simulink model "zawieszenie_samochodu"  (R2021b)
settings: Solver=ode4  StartTime=0.0  StopTime=10.0  FixedStep=1/1000  RelTol=1e-3
values from neighbouring files (symbols this model uses):
  A = [0 0 1 0; 0 0 0 1; -(k1 + k2)/m1 k2/m1 -(c1 + c2)/m1 c2/m1; k2/m2 -k2/m2 c2/m2 -c2/m2]    [workspace.m]
  B = [(c1/m1); 0; (k1/m1) - ((c1 + c2)*c1)/(m1*m1); (c1*c2)/(m1*m2)]    [workspace.m]
  C = eye(4,4)    [workspace.m]
  c1 = 100    [workspace.m]
  c2 = 2000    [workspace.m]
  D = [0; 0; 0; 0]    [workspace.m]
  k1 = 370000    [workspace.m]
  k2 = 35000    [workspace.m]
  m1 = 90    [workspace.m]
  m2 = 600    [workspace.m]
settings Model: Creator=jpawl  LastModifiedBy=jpawl

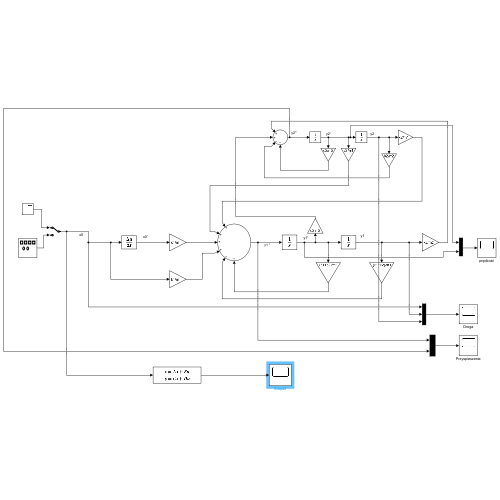
[thumbnail: Simulink's stored preview of the top-level diagram]
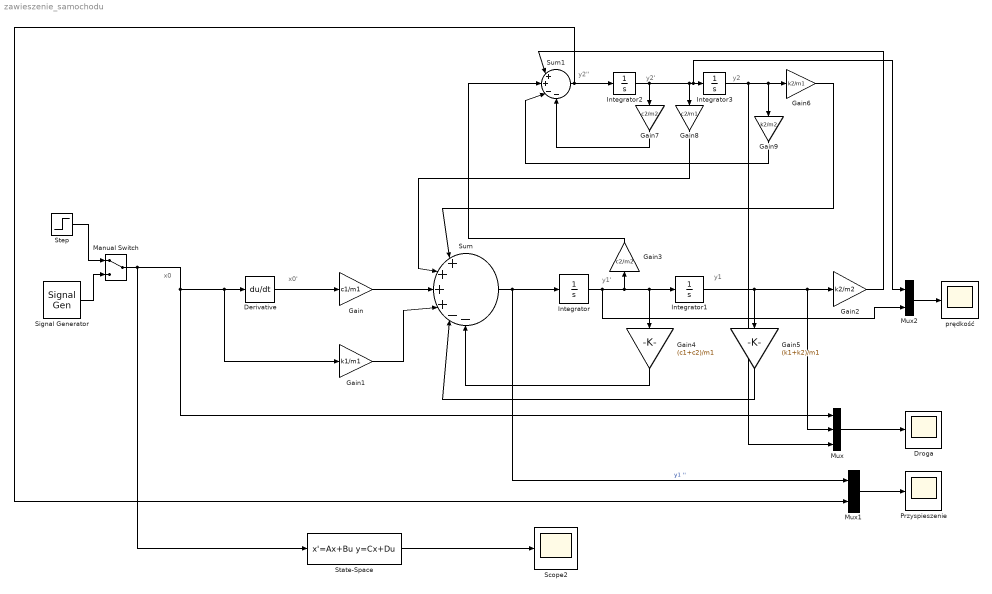
== system zawieszenie_samochodu ==
  note: y2
  note: y2'
  note: x0'
  note: x0
  note: y2''
  note: y1
  note: y1'
  Derivative : Derivative
  Droga : Scope
  Gain : Gain  Gain=c1/m1
  Gain1 : Gain  Gain=k1/m1
  Gain2 : Gain  Gain=k2/m2
  Gain3 : Gain  Gain=c2/m2
  Gain4 : Gain  Gain=(c1+c2)/m1
  Gain5 : Gain  Gain=(k1+k2)/m1
  Gain6 : Gain  Gain=k2/m1
  Gain7 : Gain  Gain=c2/m2
  Gain8 : Gain  Gain=c2/m1
  Gain9 : Gain  Gain=k2/m2
  Integrator{,1..3} (4 alike) : Integrator
  Manual Switch : ManualSwitch
  Mux : Mux  Inputs=3
  Mux1 : Mux  Inputs=2
  Mux2 : Mux  Inputs=2
  Przyspieszenie : Scope
  Scope2 : Scope
  Signal Generator : SignalGenerator  Units=rad/sec
  State-Space : StateSpace  A=A  B=B  C=C  D=D  InitialCondition=0
  Step : Step  SampleTime=0
  Sum : Sum  Inputs=|++++--
  Sum1 : Sum  Inputs=|++--
  prędkość : Scope
  wires:
  Manual Switch/1 -> State-Space/1, Mux/1, Gain1/1, Derivative/1
  Derivative/1 -> Gain/1
  Gain/1 -> Sum/3
  Gain1/1 -> Sum/4
  Sum/1 -> Mux1/1, Integrator/1  "y1 ''"
  Integrator/1 -> Mux2/2, Gain3/1, Gain4/1, Integrator1/1
  Mux/1 -> Droga/1
  Gain4/1 -> Sum/6
  Integrator1/1 -> Gain5/1, Mux/2, Gain2/1
  Gain5/1 -> Sum/5
  Gain3/1 -> Sum1/2
  Integrator2/1 -> Mux2/1, Integrator3/1, Gain8/1, Gain7/1
  Integrator3/1 -> Mux/3, Gain9/1, Gain6/1
  Gain6/1 -> Sum/1
  Gain7/1 -> Sum1/4
  Gain8/1 -> Sum/2
  Gain2/1 -> Sum1/1
  Gain9/1 -> Sum1/3
  Step/1 -> Manual Switch/1
  Signal Generator/1 -> Manual Switch/2
  Mux1/1 -> Przyspieszenie/1
  Sum1/1 -> Integrator2/1, Mux1/2
  State-Space/1 -> Scope2/1
  Mux2/1 -> prędkość/1
